simulink model "paper1_cs"  (R2021b)
settings: Solver=ode4  StartTime=0.0  StopTime=120  FixedStep=1/20  RelTol=1e-3
PreLoadFcn:
  | mbxruntime.callbacks.PreLoadFcn(bdroot);
PostLoadFcn:
  | mbxruntime.callbacks.PostLoadFcn(bdroot);
InitFcn:
  | mbxruntime.callbacks.InitFcn(bdroot);
StartFcn:
  | mbxruntime.callbacks.StartFcn(bdroot);
StopFcn:
  | mbxruntime.callbacks.StopFcn(bdroot);
model workspace (MAT data in the model file):
  mbox_table : object (value not decoded)
  model_closed = 0
  sim_status = 0
undefined symbols (not defined in the file): DiscIntNeverNeededParam
libraries: PreScanSimulinkLibrary x12, Solver_SF x6, simulink x1
(part 1 of 3)
CloseFcn:
  | mbxruntime.callbacks.CloseFcn(bdroot);
settings Model: Creator=PRESCAN  LastModifiedBy=Neutrin
settings SolverCC: AlgebraicLoopSolver=TrustRegion
settings DataIOCC: LimitDataPoints=on  SaveFormat=Array  SignalLoggingSaveFormat=ModelDataLogs  ReturnWorkspaceOutputs=off
settings OptimizationCC: ExpressionDepthLimit=2147483647  InitFltsAndDblsToZero=on  LifeSpan=inf
settings DebuggingCC: SaveWithParameterizedLinksMsg=none  UnderspecifiedInitializationDetection=Classic  MergeDetectMultiDrivingBlocksExec=none  SignalResolutionControl=TryResolveAllWithWarning  MultiTaskDSMMsg=warning  MultiTaskCondExecSysMsg=none  FcnCallInpInsideContextMsg=warning  StateNameClashWarn=warning  SFUnexpectedBacktrackingDiag=warning  SFNoUnconditionalDefaultTransitionDiag=warning  SFExecutionAtInitializationDiag=none  SFMachineParentedDataDiag=warning  ArithmeticOperatorsInVariantConditions=warning
settings HardwareCC: ProdBitPerPointer=32  ProdBitPerSizeT=32  ProdBitPerPtrDiffT=32  ProdLargestAtomicFloat=None  ProdIntDivRoundTo=Undefined  ProdEndianess=Unspecified  ProdWordSize=32  ProdHWDeviceType=32-bit Generic
settings ModelReferenceCC: UpdateModelReferenceTargets=IfOutOfDate  PropagateSignalLabelsOutOfModel=off
settings SFSimCC: SimUseLocalCustomCode=off  SimParseCustomCode=off  CustomCodeUndefinedFunction=UseInterfaceOnly
settings SFSimCC: SimCustomHeaderCode=|
  | #include "prescan.h"
  | #include "prescan_platform.h"
settings RTWCC: RTWUseLocalCustomCode=off
settings CodeAppCC: StateflowObjectComments=on
settings GRTTargetCC: TargetFcnLib=ansi_tfl_tmw.mat  TargetLangStandard=C89/C90 (ANSI)  CombineOutputUpdateFcns=off  GRTInterface=on
settings ConfigComp: CovMetricSettings=dw  CovSaveCumulativeToWorkspaceVar=on  CovSaveSingleToWorkspaceVar=on  CovExternalEMLEnable=off

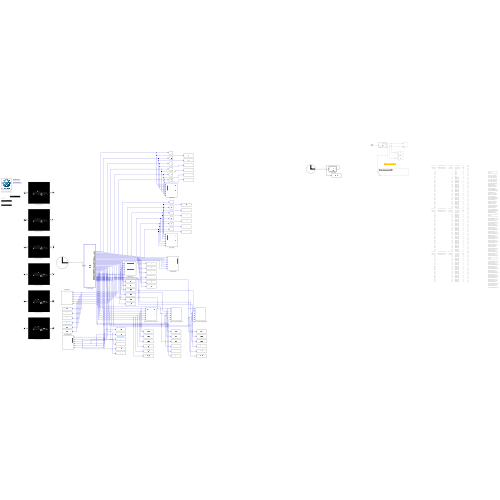
[thumbnail: Simulink's stored preview of the top-level diagram]
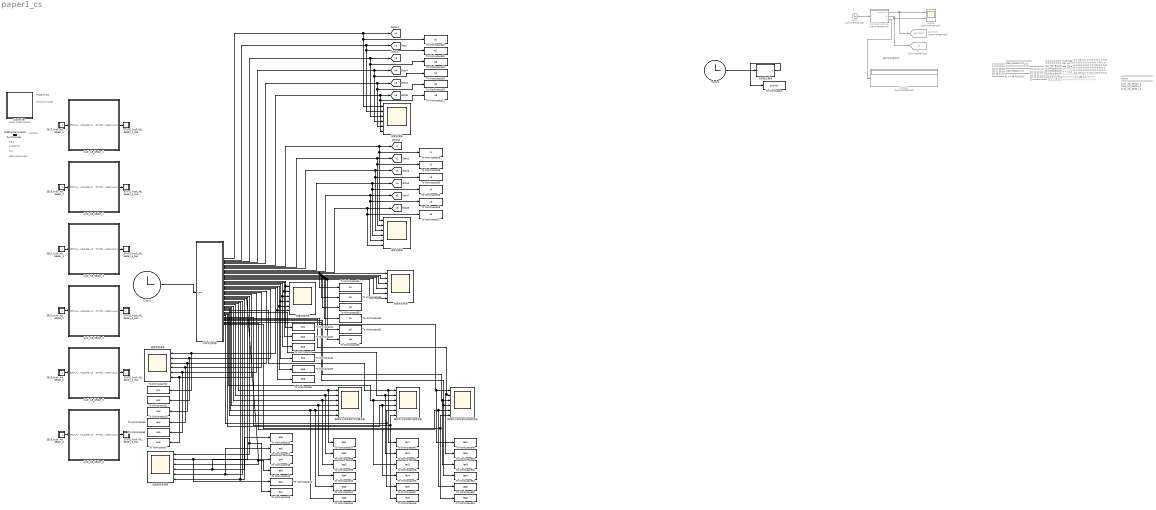
== system paper1_cs ==
  note: 虚拟领导者模块
  note: Regenerate
  note: Simulink Mode
  note: Open Useful Blocks
  note: 8.5.0
  note: Version:
  note: Author(s):
  note: N.A.
  note: Descriptive text:
  note: ======
      | Num ID
      | ======
      | 3
      | 11
      | 12
      | 13
      | 14
      | 15
      | 17
      | 19
      | 18
      | 25
      | 26
      | 27
      | 28
      | 29
      | 30
      | 32
      | 33
      | 34
      | 35
      | 36
      | 37
      | 38
      | 39
      | 40
      | 41
      | 42
      | 43
      | 44
      | 45
      | 46
      | ======
      | Num ID
      | ======
      | 31
      | 47
      | 48
      | 49
      | 50
      | 51
      | 52
      | 53
      | 54
      | 55
      | 56
      | 57
      | 58
      | 59
      | 60
      | 61
      | 62
      | 63
      | 64
      | 65
      | 66
      | 24
      | 67
      | 68
      | 20
      | 21
      | 22
      | 69
      | 70
      | 71
      | ======
      | Num ID
      | ======
      | 72
      | 73
      | 74
      | 75
      | 76
      | 77
      | 78
      | 79
      | 80
      | 81
      | 82
      | 83
      | 84
      | 85
      | 86
      | 87
      | 88
      | 89
      | 90
      | 91
      | 92
  note: =============
      | OBU-Beacon ID
      | =============
      |
      |
      |
      |
      |
      |
      |
      |
      |
      |
      |
      |
      |
      |
      |
      |
      |
      |
      |
      |
      |
      |
      |
      |
      |
      |
      |
      |
      |
      |
      | =============
      | OBU-Beacon ID
      | =============
      |
      |
      |
      |
      |
      |
      |
      |
      |
      |
      |
      |
      |
      |
      |
      |
      |
      |
      |
      |
      |
      |
      |
      |
      |
      |
      |
      |
      |
      |
      | =============
      | OBU-Beacon ID
      | =============
  note: =======
      | Type ID
      | =======
      | 1
      | 1
      | 1
      | 1
      | 1
      | 1
      | 12
      | 12
      | 12
      | 12
      | 12
      | 12
      | 12
      | 12
      | 12
      | 12
      | 12
      | 12
      | 12
      | 12
      | 12
      | 12
      | 12
      | 12
      | 12
      | 12
      | 12
      | 12
      | 12
      | 12
      | =======
      | Type ID
      | =======
      | 12
      | 12
      | 12
      | 12
      | 12
      | 12
      | 12
      | 12
      | 12
      | 12
      | 12
      | 12
      | 12
      | 12
      | 12
      | 12
      | 12
      | 12
      | 12
      | 12
      | 12
      | 12
      | 12
      | 12
      | 12
      | 12
      | 12
      | 12
      | 12
      | 12
      | =======
      | Type ID
      | =======
      | 12
      | 12
      | 12
      | 12
      | 12
      | 12
      | 12
      | 12
      | 12
      | 12
      | 12
      | 12
      | 12
      | 12
      | 12
      | 12
      | 12
      | 12
      | 12
      | 12
      | 12
  note: ========
      | Type Tag
      | ========
      | Car
      | Car
      | Car
      | Car
      | Car
      | Car
      | Building
      | Building
      | Building
      | Building
      | Building
      | Building
      | Building
      | Building
      | Building
      | Building
      | Building
      | Building
      | Building
      | Building
      | Building
      | Building
      | Building
      | Building
      | Building
      | Building
      | Building
      | Building
      | Building
      | Building
      | ========
      | Type Tag
      | ========
      | Building
      | Building
      | Building
      | Building
      | Building
      | Building
      | Building
      | Building
      | Building
      | Building
      | Building
      | Building
      | Building
      | Building
      | Building
      | Building
      | Building
      | Building
      | Building
      | Building
      | Building
      | Building
      | Building
      | Building
      | Building
      | Building
      | Building
      | Building
      | Building
      | Building
      | ========
      | Type Tag
      | ========
      | Building
      | Building
      | Building
      | Building
      | Building
      | Building
      | Building
      | Building
      | Building
      | Building
      | Building
      | Building
      | Building
      | Building
      | Building
      | Building
      | Building
      | Building
      | Building
      | Building
      | Building
  note: ==
      | SD
      | ==
      | Y
      | Y
      | Y
      | Y
      | Y
      | Y
      | Y
      | Y
      | Y
      | Y
      | Y
      | Y
      | Y
      | Y
      | Y
      | Y
      | Y
      | Y
      | Y
      | Y
      | Y
      | Y
      | Y
      | Y
      | Y
      | Y
      | Y
      | Y
      | Y
      | Y
      | ==
      | SD
      | ==
      | Y
      | Y
      | Y
      | Y
      | Y
      | Y
      | Y
      | Y
      | Y
      | Y
      | Y
      | Y
      | Y
      | Y
      | Y
      | Y
      | Y
      | Y
      | Y
      | Y
      | Y
      | Y
      | Y
      | Y
      | Y
      | Y
      | Y
      | Y
      | Y
      | Y
      | ==
      | SD
      | ==
      | Y
      | Y
      | Y
      | Y
      | Y
      | Y
      | Y
      | Y
      | Y
      | Y
      | Y
      | Y
      | Y
      | Y
      | Y
      | Y
      | Y
      | Y
      | Y
      | Y
      | Y
  note: ==
      | CD
      | ==
      | N
      | N
      | N
      | N
      | N
      | N
      | N
      | N
      | N
      | N
      | N
      | N
      | N
      | N
      | N
      | N
      | N
      | N
      | N
      | N
      | N
      | N
      | N
      | N
      | N
      | N
      | N
      | N
      | N
      | N
      | ==
      | CD
      | ==
      | N
      | N
      | N
      | N
      | N
      | N
      | N
      | N
      | N
      | N
      | N
      | N
      | N
      | N
      | N
      | N
      | N
      | N
      | N
      | N
      | N
      | N
      | N
      | N
      | N
      | N
      | N
      | N
      | N
      | N
      | ==
      | CD
      | ==
      | N
      | N
      | N
      | N
      | N
      | N
      | N
      | N
      | N
      | N
      | N
      | N
      | N
      | N
      | N
      | N
      | N
      | N
      | N
      | N
      | N
  note: ================
      | Name
      | ================
      | Audi_A8_Sedan_1
      | Audi_A8_Sedan_2
      | Audi_A8_Sedan_3
      | Audi_A8_Sedan_4
      | Audi_A8_Sedan_5
      | Audi_A8_Sedan_6
      | ApartmentBuilding_1
      | HouseModern_1
      | OfficeGreenTall_1
      | OfficeGreenTall_3
      | HouseModern_3
      | ApartmentBuilding_3
      | ApartmentBuilding_4
      | HouseModern_4
      | OfficeGreenTall_4
      | OfficeGreenTall_5
      | HouseModern_5
      | ApartmentBuilding_5
      | ApartmentBuilding_6
      | HouseModern_6
      | OfficeGreenTall_6
      | OfficeGreenTall_7
      | HouseModern_7
      | ApartmentBuilding_7
      | OfficeGreenTall_8
      | HouseModern_8
      | ApartmentBuilding_8
      | ApartmentBuilding_9
      | HouseModern_9
      | OfficeGreenTall_9
      | ================
      | Name
      | ================
      | ApartmentBuilding_10
      | HouseModern_10
      | OfficeGreenTall_10
      | ApartmentBuilding_11
      | HouseModern_11
      | OfficeGreenTall_11
      | ApartmentBuilding_12
      | HouseModern_12
      | OfficeGreenTall_12
      | ApartmentBuilding_13
      | HouseModern_13
      | OfficeGreenTall_13
      | ApartmentBuilding_14
      | HouseModern_14
      | OfficeGreenTall_14
      | ApartmentBuilding_15
      | HouseModern_15
      | OfficeGreenTall_15
      | ApartmentBuilding_16
      | HouseModern_16
      | OfficeGreenTall_16
      | OfficeGreenTall_2
      | HouseModern_2
      | ApartmentBuilding_2
      | OfficeGreenTall_17
      | HouseModern_17
      | ApartmentBuilding_17
      | OfficeGreenTall_18
      | HouseModern_18
      | ApartmentBuilding_18
      | ================
      | Name
      | ================
      | ApartmentBuilding_19
      | HouseModern_19
      | OfficeGreenTall_19
      | ApartmentBuilding_20
      | HouseModern_20
      | OfficeGreenTall_20
      | ApartmentBuilding_21
      | HouseModern_21
      | OfficeGreenTall_21
      | ApartmentBuilding_22
      | HouseModern_22
      | OfficeGreenTall_22
      | ApartmentBuilding_23
      | HouseModern_23
      | OfficeGreenTall_23
      | OfficeGreenTall_24
      | HouseModern_24
      | ApartmentBuilding_24
      | OfficeGreenTall_25
      | HouseModern_25
      | ApartmentBuilding_25
  Audi_A8_Sedan_1 : Subsystem  Tag=WorldObjectSubSystem  InitFcn=UniqueId = '64';
      mask init:
      | modelPath = GenericModelHelper.getGenericModelFilePath('ModelDepo','Vehicles\Audi_A8\Audi_A8.pgmb','d771622804618130053427da08a6d484');imagePath = GenericModelHelper.getCompilationPicture(modelPath, 'Audi_A8_HighPoly.png');
      mask Display: image(imread(imagePath));color('white');text(0, 0, ' ID=3\n')
  Audi_A8_Sedan_2 : Subsystem  Tag=WorldObjectSubSystem  InitFcn=UniqueId = '65';
      mask init: same as paper1_cs/Audi_A8_Sedan_1
      mask Display: image(imread(imagePath));color('white');text(0, 0, ' ID=11\n')
  Audi_A8_Sedan_3 : Subsystem  Tag=WorldObjectSubSystem  InitFcn=UniqueId = '66';
      mask init: same as paper1_cs/Audi_A8_Sedan_1
      mask Display: image(imread(imagePath));color('white');text(0, 0, ' ID=12\n')
  Audi_A8_Sedan_4 : Subsystem  Tag=WorldObjectSubSystem  InitFcn=UniqueId = '67';
      mask init: same as paper1_cs/Audi_A8_Sedan_1
      mask Display: image(imread(imagePath));color('white');text(0, 0, ' ID=13\n')
  Audi_A8_Sedan_5 : Subsystem  Tag=WorldObjectSubSystem  InitFcn=UniqueId = '68';
      mask init: same as paper1_cs/Audi_A8_Sedan_1
      mask Display: image(imread(imagePath));color('white');text(0, 0, ' ID=14\n')
  Audi_A8_Sedan_6 : Subsystem  Tag=WorldObjectSubSystem  InitFcn=UniqueId = '69';
      mask init: same as paper1_cs/Audi_A8_Sedan_1
      mask Display: image(imread(imagePath));color('white');text(0, 0, ' ID=15\n')
  Clock : Clock  Commented=on
  Clock1 : Clock
  Clock2 : Clock
  Controller : Subsystem  Description=FAA03037B41319C220BECF1B5D4CC9BCB680DCDF6B1D9774133C0D9A14409DD5  Priority=-1  LoadFcn=load PreScanControllerData  mask(PreScan Simulation Controller){prescanversion='8.5.0', ModelReferencing=off, TimeStep=1/20, ControlMode=0, PreScanExecutionMode=on, ControllerCount=0, ControllerIndex=0, ControllerOptions=''}
      mask prompts: prescanversion "PreScan Version"; ModelReferencing "Use Model Referencing"; TimeStep "Upload Period [s]"; ControlMode "Control Mode"; PreScanExecutionMode "Execution Mode"; ControllerCount "Controller Count"; ControllerIndex "Controller Index"; ControllerOptions "Controller Options"
      mask help:
      | Please do not remove this block from the compilation sheet,
      | as it connects the model to the PreScan environment.
      mask init:
      | model = bdroot(gcb);
      | ExperimentFile = mbxruntime.findExperimentFile(model,true); %relative path
      | 
      | [d1, d2, d3, prescandata] = prescan_Settings();
      | ModelDepo = fullfile(prescandata,'ModelDepo'); 
      | 
      | RTmode = mbxruntime.getRTMode(model);
      | 
      | SimulationMode = get_param(bdroot,'SimulationMode');
      | if strcmp(SimulationMode, 'rapid-accelerator')
      |     SimulationMode = 'external';
      | end
      | TargetName = get_param(bdroot,'SystemTargetFile');
      settings: ModelCloseFcn=assignin('base',['model_closed_' bdroot],true);
      mask Help: eval('openHelp(812)')
      mask Display: image(imread('prescanlogo.ico'))
  Display : Display  Commented=on
  MATLAB Function : MATLAB Function  Commented=on  TreatAsAtomicUnit=on
  PreScanTerminator : Subsystem  Tag=PreScanTerminator  Priority=999  LoadFcn=load PrescanTerminatorData  mask(PreScan Simulation Terminator){TimeStep=1/20}
      mask prompts: TimeStep "Upload Period [s]"
      mask help:
      | Please do not remove this block from the compilation sheet as it
      | connects the model to the PreScan environment.
      mask Help: eval('openHelp(812)')
      mask Display: image(imread('prescanlogo.ico'))
  SELF_Audi_A8_Sedan_1 : Subsystem  Tag=sensor/SelfPort  Priority=3  LoadFcn=load('PreScanSelfSensorData.mat')  mask(PreScan Source Block: SELF){}
      mask help:
      | The SELF port shows (state) information of the actor itself. The outputs are position in the experiment's axis system and the GPS coordinates, and the object's absolute velocity and compass heading.
      |
      | For more information, please click Help.
      settings: OpenFcn=open_system([gcb '/Sensor'],'mask')
      mask Help: eval('openHelp(462)')
      mask Display: image(imread('GPS.png'))
  SELF_Audi_A8_Sedan_2 : Subsystem  Tag=sensor/SelfPort  Priority=3  LoadFcn=load('PreScanSelfSensorData.mat')  mask(PreScan Source Block: SELF){}
      mask help:
      | The SELF port shows (state) information of the actor itself. The outputs are position in the experiment's axis system and the GPS coordinates, and the object's absolute velocity and compass heading.
      |
      | For more information, please click Help.
      settings: OpenFcn=open_system([gcb '/Sensor'],'mask')
      mask Help: eval('openHelp(462)')
      mask Display: image(imread('GPS.png'))
  SELF_Audi_A8_Sedan_3 : Subsystem  Tag=sensor/SelfPort  Priority=3  LoadFcn=load('PreScanSelfSensorData.mat')  mask(PreScan Source Block: SELF){}
      mask help:
      | The SELF port shows (state) information of the actor itself. The outputs are position in the experiment's axis system and the GPS coordinates, and the object's absolute velocity and compass heading.
      |
      | For more information, please click Help.
      settings: OpenFcn=open_system([gcb '/Sensor'],'mask')
      mask Help: eval('openHelp(462)')
      mask Display: image(imread('GPS.png'))
  SELF_Audi_A8_Sedan_4 : Subsystem  Tag=sensor/SelfPort  Priority=3  LoadFcn=load('PreScanSelfSensorData.mat')  mask(PreScan Source Block: SELF){}
      mask help:
      | The SELF port shows (state) information of the actor itself. The outputs are position in the experiment's axis system and the GPS coordinates, and the object's absolute velocity and compass heading.
      |
      | For more information, please click Help.
      settings: OpenFcn=open_system([gcb '/Sensor'],'mask')
      mask Help: eval('openHelp(462)')
      mask Display: image(imread('GPS.png'))
  SELF_Audi_A8_Sedan_5 : Subsystem  Tag=sensor/SelfPort  Priority=3  LoadFcn=load('PreScanSelfSensorData.mat')  mask(PreScan Source Block: SELF){}
      mask help:
      | The SELF port shows (state) information of the actor itself. The outputs are position in the experiment's axis system and the GPS coordinates, and the object's absolute velocity and compass heading.
      |
      | For more information, please click Help.
      settings: OpenFcn=open_system([gcb '/Sensor'],'mask')
      mask Help: eval('openHelp(462)')
      mask Display: image(imread('GPS.png'))
  SELF_Audi_A8_Sedan_6 : Subsystem  Tag=sensor/SelfPort  Priority=3  LoadFcn=load('PreScanSelfSensorData.mat')  mask(PreScan Source Block: SELF){}
      mask help:
      | The SELF port shows (state) information of the actor itself. The outputs are position in the experiment's axis system and the GPS coordinates, and the object's absolute velocity and compass heading.
      |
      | For more information, please click Help.
      settings: OpenFcn=open_system([gcb '/Sensor'],'mask')
      mask Help: eval('openHelp(462)')
      mask Display: image(imread('GPS.png'))
  STATE_Audi_A8_Sedan_1_bus : Subsystem  Tag=actuator/StatePort  Priority=0  LoadFcn=load('PreScanStateActuatorData.mat')  mask(PreScan Sink Block: State){}
      mask help:
      | The Actor State contains a vector signal of size (9x1), containing the following signals:
      |
      | -  Position    	(x,y,z)             	[m]
      | -  Velocity    	(vx,vy,vz)         	[m/s]
      | -  Angles       	(Roll, Pitch, Yaw)	[rad]
      |
      | The Actor state is defined in the global axis system.
      | The state is superponed on the Initial position defined in the GUI.
      |
      | For more information, please click Help.
      settings: OpenFcn=open_system([gcb '/Actuator'],'mask')
      mask Help: eval('openHelp(222)')
      mask Display: image(imread('State.png'))
  STATE_Audi_A8_Sedan_2_bus : Subsystem  Tag=actuator/StatePort  Priority=0  LoadFcn=load('PreScanStateActuatorData.mat')  mask(PreScan Sink Block: State){}
      mask help:
      | The Actor State contains a vector signal of size (9x1), containing the following signals:
      |
      | -  Position    	(x,y,z)             	[m]
      | -  Velocity    	(vx,vy,vz)         	[m/s]
      | -  Angles       	(Roll, Pitch, Yaw)	[rad]
      |
      | The Actor state is defined in the global axis system.
      | The state is superponed on the Initial position defined in the GUI.
      |
      | For more information, please click Help.
      settings: OpenFcn=open_system([gcb '/Actuator'],'mask')
      mask Help: eval('openHelp(222)')
      mask Display: image(imread('State.png'))
  STATE_Audi_A8_Sedan_3_bus : Subsystem  Tag=actuator/StatePort  Priority=0  LoadFcn=load('PreScanStateActuatorData.mat')  mask(PreScan Sink Block: State){}
      mask help:
      | The Actor State contains a vector signal of size (9x1), containing the following signals:
      |
      | -  Position    	(x,y,z)             	[m]
      | -  Velocity    	(vx,vy,vz)         	[m/s]
      | -  Angles       	(Roll, Pitch, Yaw)	[rad]
      |
      | The Actor state is defined in the global axis system.
      | The state is superponed on the Initial position defined in the GUI.
      |
      | For more information, please click Help.
      settings: OpenFcn=open_system([gcb '/Actuator'],'mask')
      mask Help: eval('openHelp(222)')
      mask Display: image(imread('State.png'))
  STATE_Audi_A8_Sedan_4_bus : Subsystem  Tag=actuator/StatePort  Priority=0  LoadFcn=load('PreScanStateActuatorData.mat')  mask(PreScan Sink Block: State){}
      mask help:
      | The Actor State contains a vector signal of size (9x1), containing the following signals:
      |
      | -  Position    	(x,y,z)             	[m]
      | -  Velocity    	(vx,vy,vz)         	[m/s]
      | -  Angles       	(Roll, Pitch, Yaw)	[rad]
      |
      | The Actor state is defined in the global axis system.
      | The state is superponed on the Initial position defined in the GUI.
      |
      | For more information, please click Help.
      settings: OpenFcn=open_system([gcb '/Actuator'],'mask')
      mask Help: eval('openHelp(222)')
      mask Display: image(imread('State.png'))
  STATE_Audi_A8_Sedan_5_bus : Subsystem  Tag=actuator/StatePort  Priority=0  LoadFcn=load('PreScanStateActuatorData.mat')  mask(PreScan Sink Block: State){}
      mask help:
      | The Actor State contains a vector signal of size (9x1), containing the following signals:
      |
      | -  Position    	(x,y,z)             	[m]
      | -  Velocity    	(vx,vy,vz)         	[m/s]
      | -  Angles       	(Roll, Pitch, Yaw)	[rad]
      |
      | The Actor state is defined in the global axis system.
      | The state is superponed on the Initial position defined in the GUI.
      |
      | For more information, please click Help.
      settings: OpenFcn=open_system([gcb '/Actuator'],'mask')
      mask Help: eval('openHelp(222)')
      mask Display: image(imread('State.png'))
  STATE_Audi_A8_Sedan_6_bus : Subsystem  Tag=actuator/StatePort  Priority=0  LoadFcn=load('PreScanStateActuatorData.mat')  mask(PreScan Sink Block: State){}
      mask help:
      | The Actor State contains a vector signal of size (9x1), containing the following signals:
      |
      | -  Position    	(x,y,z)             	[m]
      | -  Velocity    	(vx,vy,vz)         	[m/s]
      | -  Angles       	(Roll, Pitch, Yaw)	[rad]
      |
      | The Actor state is defined in the global axis system.
      | The state is superponed on the Initial position defined in the GUI.
      |
      | For more information, please click Help.
      settings: OpenFcn=open_system([gcb '/Actuator'],'mask')
      mask Help: eval('openHelp(222)')
      mask Display: image(imread('State.png'))
  Scope : Scope  Commented=on  NumInputPorts=2
  Synchronizer : Subsystem  Tag=PreScanSynchronizer  Priority=1  LoadFcn=load PrescanSynchronizeData  mask(PreScan Simulation Core Block){TimeStep=1/20}
      mask prompts: TimeStep "Timestep [s]"
      mask help:
      | Please do not remove this block from the PreScan compilation sheet,
      | as it contains essential configuration parameters for a PreScan simulation.
      settings: DeleteFcn=PreScanBlockDeleteFcn;
      mask Display: image(imread('prescanlogo.ico'))
  To Workspace : ToWorkspace  VariableName=simout  SaveFormat=Timeseries  SampleTime=-1
  To Workspace1 : ToWorkspace  VariableName=ep1  SaveFormat=Timeseries  SampleTime=-1
  To Workspace10 : ToWorkspace  VariableName=ev3  SaveFormat=Timeseries  SampleTime=-1
  To Workspace11 : ToWorkspace  VariableName=ev2  SaveFormat=Timeseries  SampleTime=-1
  To Workspace12 : ToWorkspace  VariableName=ev1  SaveFormat=Timeseries  SampleTime=-1
  To Workspace13 : ToWorkspace  VariableName=ea3  SaveFormat=Timeseries  SampleTime=-1
  To Workspace14 : ToWorkspace  VariableName=ea2  SaveFormat=Timeseries  SampleTime=-1
  To Workspace15 : ToWorkspace  VariableName=ea1  SaveFormat=Timeseries  SampleTime=-1
  To Workspace16 : ToWorkspace  VariableName=ea6  SaveFormat=Timeseries  SampleTime=-1
  To Workspace17 : ToWorkspace  VariableName=ea5  SaveFormat=Timeseries  SampleTime=-1
  To Workspace18 : ToWorkspace  VariableName=ea4  SaveFormat=Timeseries  SampleTime=-1
  To Workspace19 : ToWorkspace  VariableName=p4  SaveFormat=Timeseries  SampleTime=-1
  To Workspace2 : ToWorkspace  VariableName=ep2  SaveFormat=Timeseries  SampleTime=-1
  To Workspace20 : ToWorkspace  VariableName=p5  SaveFormat=Timeseries  SampleTime=-1
  To Workspace21 : ToWorkspace  VariableName=p6  SaveFormat=Timeseries  SampleTime=-1
  To Workspace22 : ToWorkspace  VariableName=p1  SaveFormat=Timeseries  SampleTime=-1
  To Workspace23 : ToWorkspace  VariableName=p2  SaveFormat=Timeseries  SampleTime=-1
  To Workspace24 : ToWorkspace  VariableName=p3  SaveFormat=Timeseries  SampleTime=-1
  To Workspace25 : ToWorkspace  VariableName=v4  SaveFormat=Timeseries  SampleTime=-1
  To Workspace26 : ToWorkspace  VariableName=v5  SaveFormat=Timeseries  SampleTime=-1
  To Workspace27 : ToWorkspace  VariableName=v6  SaveFormat=Timeseries  SampleTime=-1
  To Workspace28 : ToWorkspace  VariableName=v1  SaveFormat=Timeseries  SampleTime=-1
  To Workspace29 : ToWorkspace  VariableName=v2  SaveFormat=Timeseries  SampleTime=-1
  To Workspace3 : ToWorkspace  VariableName=ep3  SaveFormat=Timeseries  SampleTime=-1
  To Workspace30 : ToWorkspace  VariableName=v3  SaveFormat=Timeseries  SampleTime=-1
  To Workspace31 : ToWorkspace  VariableName=a4  SaveFormat=Timeseries  SampleTime=-1
  To Workspace32 : ToWorkspace  VariableName=a5  SaveFormat=Timeseries  SampleTime=-1
  To Workspace33 : ToWorkspace  VariableName=a6  SaveFormat=Timeseries  SampleTime=-1
  To Workspace34 : ToWorkspace  VariableName=a1  SaveFormat=Timeseries  SampleTime=-1
  To Workspace35 : ToWorkspace  VariableName=a2  SaveFormat=Timeseries  SampleTime=-1
  To Workspace36 : ToWorkspace  VariableName=a3  SaveFormat=Timeseries  SampleTime=-1
  To Workspace37 : ToWorkspace  VariableName=lep1  SaveFormat=Timeseries  SampleTime=-1
  To Workspace38 : ToWorkspace  VariableName=lep2  SaveFormat=Timeseries  SampleTime=-1
  To Workspace39 : ToWorkspace  VariableName=lep3  SaveFormat=Timeseries  SampleTime=-1
  To Workspace4 : ToWorkspace  VariableName=ep4  SaveFormat=Timeseries  SampleTime=-1
  To Workspace40 : ToWorkspace  VariableName=lep4  SaveFormat=Timeseries  SampleTime=-1
  To Workspace41 : ToWorkspace  VariableName=lep5  SaveFormat=Timeseries  SampleTime=-1
  To Workspace42 : ToWorkspace  VariableName=lep6  SaveFormat=Timeseries  SampleTime=-1
  To Workspace43 : ToWorkspace  VariableName=lev1  SaveFormat=Timeseries  SampleTime=-1
  To Workspace44 : ToWorkspace  VariableName=lev2  SaveFormat=Timeseries  SampleTime=-1
  To Workspace45 : ToWorkspace  VariableName=lev3  SaveFormat=Timeseries  SampleTime=-1
  To Workspace46 : ToWorkspace  VariableName=lev4  SaveFormat=Timeseries  SampleTime=-1
  To Workspace47 : ToWorkspace  VariableName=lev5  SaveFormat=Timeseries  SampleTime=-1
  To Workspace48 : ToWorkspace  VariableName=lev6  SaveFormat=Timeseries  SampleTime=-1
  To Workspace49 : ToWorkspace  VariableName=lea1  SaveFormat=Timeseries  SampleTime=-1
  To Workspace5 : ToWorkspace  VariableName=ep5  SaveFormat=Timeseries  SampleTime=-1
  To Workspace50 : ToWorkspace  VariableName=lea2  SaveFormat=Timeseries  SampleTime=-1
  To Workspace51 : ToWorkspace  VariableName=lea3  SaveFormat=Timeseries  SampleTime=-1
  To Workspace52 : ToWorkspace  VariableName=lea4  SaveFormat=Timeseries  SampleTime=-1
  To Workspace53 : ToWorkspace  VariableName=lea5  SaveFormat=Timeseries  SampleTime=-1
  To Workspace54 : ToWorkspace  VariableName=lea6  SaveFormat=Timeseries  SampleTime=-1
  To Workspace6 : ToWorkspace  VariableName=ep6  SaveFormat=Timeseries  SampleTime=-1
  To Workspace7 : ToWorkspace  VariableName=ev6  SaveFormat=Timeseries  SampleTime=-1
  To Workspace8 : ToWorkspace  VariableName=ev5  SaveFormat=Timeseries  SampleTime=-1
  To Workspace9 : ToWorkspace  VariableName=ev4  SaveFormat=Timeseries  SampleTime=-1
  position0 : Goto  Commented=on  GotoTag=position0  TagVisibility=global
  v0 : Goto  Commented=on  GotoTag=v0  TagVisibility=global
  位置监视器 : Scope  NumInputPorts=6
  位置观测误差 : Scope  NumInputPorts=6
  分布式控制器 : MATLAB Function  TreatAsAtomicUnit=on
  加速度监视器 : Scope  NumInputPorts=6
  加速度观测误差 : Scope  NumInputPorts=6
  时序验证模块 : MATLAB Function  TreatAsAtomicUnit=on
  跟随车与领导者的加速度误差 : Scope  NumInputPorts=6
  跟随车与领导者的状位置误差 : Scope  NumInputPorts=6
  跟随车与领导者的速度误差 : Scope  NumInputPorts=6
  速度监视器 : Scope  NumInputPorts=6
  速度观测误差 : Scope  NumInputPorts=6
  tag scope: v1=global, v2=global, v3=global, v4=global, v5=global, v6=global, x1=global, x2=global, x3=global, x4=global, x5=global, x6=global
  wires:
  Clock/1 -> MATLAB Function/1("t ")
  MATLAB Function/2(v0) -> v0/1, Scope/2
  MATLAB Function/1(position0) -> position0/1, Scope/1
  MATLAB Function/3(t) -> Display/1
  Clock1/1 -> 分布式控制器/1(time)
  时序验证模块/1(y) -> To Workspace/1
  Clock2/1 -> 时序验证模块/1(t)
  Audi_A8_Sedan_1/1(STATE_Audi_A8_Sedan_1_bus) -> STATE_Audi_A8_Sedan_1_bus/1(STATE_Audi_A8_Sedan_1_bus)
  SELF_Audi_A8_Sedan_1/1(SELF_Audi_A8_Sedan_1) -> Audi_A8_Sedan_1/1(SELF_Audi_A8_Sedan_1)
  Audi_A8_Sedan_2/1(STATE_Audi_A8_Sedan_2_bus) -> STATE_Audi_A8_Sedan_2_bus/1(STATE_Audi_A8_Sedan_2_bus)
  SELF_Audi_A8_Sedan_2/1(SELF_Audi_A8_Sedan_2) -> Audi_A8_Sedan_2/1(SELF_Audi_A8_Sedan_2)
  Audi_A8_Sedan_3/1(STATE_Audi_A8_Sedan_3_bus) -> STATE_Audi_A8_Sedan_3_bus/1(STATE_Audi_A8_Sedan_3_bus)
  SELF_Audi_A8_Sedan_3/1(SELF_Audi_A8_Sedan_3) -> Audi_A8_Sedan_3/1(SELF_Audi_A8_Sedan_3)
  Audi_A8_Sedan_4/1(STATE_Audi_A8_Sedan_4_bus) -> STATE_Audi_A8_Sedan_4_bus/1(STATE_Audi_A8_Sedan_4_bus)
  SELF_Audi_A8_Sedan_4/1(SELF_Audi_A8_Sedan_4) -> Audi_A8_Sedan_4/1(SELF_Audi_A8_Sedan_4)
  Audi_A8_Sedan_5/1(STATE_Audi_A8_Sedan_5_bus) -> STATE_Audi_A8_Sedan_5_bus/1(STATE_Audi_A8_Sedan_5_bus)
  SELF_Audi_A8_Sedan_5/1(SELF_Audi_A8_Sedan_5) -> Audi_A8_Sedan_5/1(SELF_Audi_A8_Sedan_5)
  Audi_A8_Sedan_6/1(STATE_Audi_A8_Sedan_6_bus) -> STATE_Audi_A8_Sedan_6_bus/1(STATE_Audi_A8_Sedan_6_bus)
  SELF_Audi_A8_Sedan_6/1(SELF_Audi_A8_Sedan_6) -> Audi_A8_Sedan_6/1(SELF_Audi_A8_Sedan_6)
  分布式控制器/1(p1) -> To Workspace22/1, 位置监视器/1, [x1]
  分布式控制器/2(p2) -> To Workspace23/1, 位置监视器/2, [x2]
  分布式控制器/3(p3) -> To Workspace24/1, 位置监视器/3, [x3]
  分布式控制器/4(p4) -> To Workspace19/1, 位置监视器/4, [x4]
  分布式控制器/5(p5) -> To Workspace20/1, 位置监视器/5, [x5]
  分布式控制器/6(p6) -> To Workspace21/1, 位置监视器/6, [x6]
  分布式控制器/7(v1) -> To Workspace28/1, 速度监视器/1, [v1]
  分布式控制器/8(v2) -> To Workspace29/1, 速度监视器/2, [v2]
  分布式控制器/9(v3) -> 速度监视器/3, To Workspace30/1, [v3]
  分布式控制器/10(v4) -> To Workspace25/1, 速度监视器/4, [v4]
  分布式控制器/11(v5) -> [v5], To Workspace26/1, 速度监视器/5
  分布式控制器/12(v6) -> To Workspace27/1, 速度监视器/6, [v6]
  分布式控制器/13(as1) -> 加速度监视器/1, To Workspace34/1
  分布式控制器/14(as2) -> To Workspace35/1, 加速度监视器/2
  分布式控制器/15(as3) -> To Workspace36/1, 加速度监视器/3
  分布式控制器/16(as4) -> To Workspace31/1, 加速度监视器/4
  分布式控制器/17(as5) -> To Workspace32/1, 加速度监视器/5
  分布式控制器/18(as6) -> To Workspace33/1, 加速度监视器/6
  分布式控制器/19(ep1) -> To Workspace1/1, 位置观测误差/1
  分布式控制器/20(ep2) -> To Workspace2/1, 位置观测误差/2
  分布式控制器/21(ep3) -> To Workspace3/1, 位置观测误差/3
  分布式控制器/22(ep4) -> To Workspace4/1, 位置观测误差/4
  分布式控制器/23(ep5) -> To Workspace5/1, 位置观测误差/5
  分布式控制器/24(ep6) -> To Workspace6/1, 位置观测误差/6
  分布式控制器/25(ev1) -> To Workspace12/1, 速度观测误差/1
  分布式控制器/26(ev2) -> To Workspace11/1, 速度观测误差/2
  分布式控制器/27(ev3) -> To Workspace10/1, 速度观测误差/3
  分布式控制器/28(ev4) -> To Workspace9/1, 速度观测误差/4
  分布式控制器/29(ev5) -> To Workspace8/1, 速度观测误差/5
  分布式控制器/30(ev6) -> To Workspace7/1, 速度观测误差/6
  分布式控制器/31(ea1) -> 加速度观测误差/1, To Workspace15/1
  分布式控制器/32(ea2) -> 加速度观测误差/2, To Workspace14/1
  分布式控制器/33(ea3) -> 加速度观测误差/3, To Workspace13/1
  分布式控制器/34(ea4) -> 加速度观测误差/4, To Workspace18/1
  分布式控制器/35(ea5) -> 加速度观测误差/5, To Workspace17/1
  分布式控制器/36(ea6) -> 加速度观测误差/6, To Workspace16/1
  分布式控制器/37(lep1) -> To Workspace37/1, 跟随车与领导者的状位置误差/1
  分布式控制器/38(lep2) -> To Workspace38/1, 跟随车与领导者的状位置误差/2
  分布式控制器/39(lep3) -> To Workspace39/1, 跟随车与领导者的状位置误差/3
  分布式控制器/40(lep4) -> To Workspace40/1, 跟随车与领导者的状位置误差/4
  分布式控制器/41(lep5) -> To Workspace42/1, To Workspace41/1, 跟随车与领导者的状位置误差/5
  分布式控制器/42(lep6) -> 跟随车与领导者的状位置误差/6
  分布式控制器/43(lev1) -> To Workspace43/1, 跟随车与领导者的速度误差/1
  分布式控制器/44(lev2) -> To Workspace44/1, 跟随车与领导者的速度误差/2
  分布式控制器/45(lev3) -> To Workspace45/1, 跟随车与领导者的速度误差/3
  分布式控制器/46(lev4) -> To Workspace46/1, 跟随车与领导者的速度误差/4
  分布式控制器/47(lev5) -> 跟随车与领导者的速度误差/5, To Workspace47/1
  分布式控制器/48(lev6) -> 跟随车与领导者的速度误差/6, To Workspace48/1
  分布式控制器/49(lea1) -> To Workspace49/1, 跟随车与领导者的加速度误差/1
  分布式控制器/50(lea2) -> To Workspace50/1, 跟随车与领导者的加速度误差/2
  分布式控制器/51(lea3) -> To Workspace51/1, 跟随车与领导者的加速度误差/3
  分布式控制器/52(lea4) -> To Workspace52/1, 跟随车与领导者的加速度误差/4
  分布式控制器/53(lea5) -> 跟随车与领导者的加速度误差/5, To Workspace53/1
  分布式控制器/54(lea6) -> To Workspace54/1, 跟随车与领导者的加速度误差/6

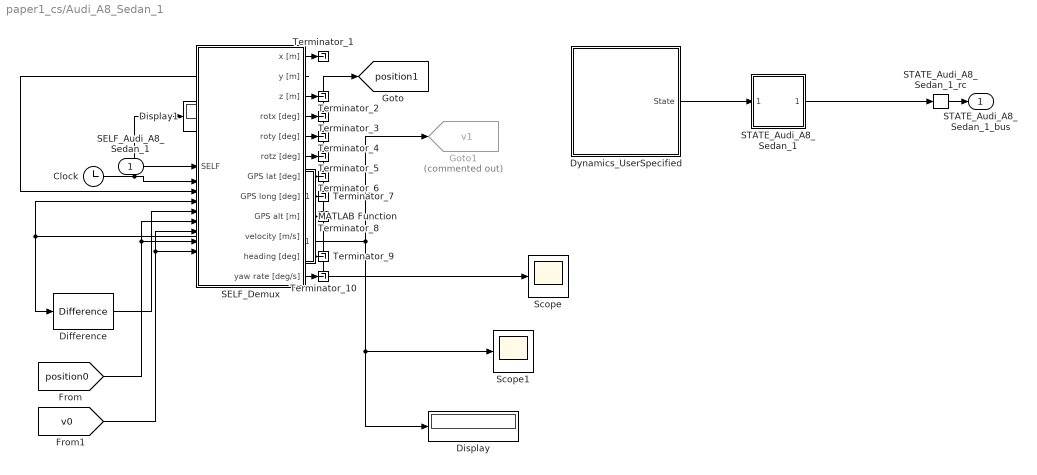
== system paper1_cs/Audi_A8_Sedan_1 ==
  SELF_Audi_A8_Sedan_1 : Inport  Tag=inport/SelfPort  OutDataTypeStr=Bus: PRESCAN_SELFSENSORDATA  PortDimensions=1  SampleTime=1/20  BusOutputAsStruct=on
  Clock : Clock
  Difference : simulink/Discrete/Difference  ICPrevInput=0.0  OutMin=[]  OutMax=[]  OutDataType=fixdt(1, 16)  OutScaling=2^-10  DoSatur=off
  Display : Display
  Display1 : Display
  Dynamics_UserSpecified : Subsystem  Tag=UserSpecified_Subsys  Description=..\..\..\DynamicMode\Extensions\Simulink\CarSim_VehicleDynamics.mdl  mask(User specified subsystem){update=off, sourcefilename=..\..\..\DynamicMode\Extensions\Simulink\CarSim_VehicleDynamics.mdl}
      mask prompts: update "Update (default: not checked)"; sourcefilename "Source file name"
      mask help:
      | A User-specified model may be selected as Controller or Dynamics of the vehicle. PreScan will copy the contents of the User-specified model into the user-specified model block.
      |
      | If update checkbox is checked the current user-specified model block will be deleted and will be REPLACED by (new) user specified model blocks. So, the current user specified model elements will be lost.
      |
      | Warning: If a new user-specified model is selected in the GUI, the user-specified model will be replaced.
      settings: DeleteFcn=PreScanBlockDeleteFcn;
      mask Help: eval('openHelp(227)')
      mask Display: userSpecifiedDynamics_mask_display();
  Goto1 : Goto  Commented=on  GotoTag=v1  TagVisibility=global
  MATLAB Function : MATLAB Function  TreatAsAtomicUnit=on
  SELF_Demux : Subsystem  Tag=demux/SelfPort  mask(PreScan Demux Block:){}
      mask help:
      | The SELF port shows (state) information of the actor itself. The outputs are position in the experiment's axis system and the GPS coordinates, and the object's absolute velocity and compass heading.
      |
      | For more information, please click Help.
      settings: DeleteFcn=PreScanBlockDeleteFcn;
      mask Help: eval('openHelp(462)')
      mask Display:
      | port_label('output',1,'x [m]')
      | port_label('output',2,'y [m]')
      | port_label('output',3,'z [m]','texmode','on')
      | port_label('output',4,'Rotx [deg]','texmode','on')
      | port_label('output',5,'Roty [deg]','texmode','on')
      | port_label('output',6,'Rotz [deg]','texmode','on')
      | port_label('output',7,'GPS lat [deg]','texmode','on')
      | port_label('output',8,'GPS long [deg]','texmode','on')
      | port_label('output',9,'GPS alt [m]','texmode','on')
      | port_label('output',10,'Velocity [m/s]')
      | port_label('output',11,'Heading [deg]')
      | port_label('output',12,'Yaw rate [deg/s]')
  STATE_Audi_A8_Sedan_1 : Subsystem  Tag=mux/StatePort  Priority=0  LoadFcn=load PrescanStateActuatorData  mask(PreScan Sink Block: State){x0=120, y0=85, z0=0.55, Roll0=0, Pitch0=0, Yaw0=0, TimeStep=1/20}
      mask prompts: x0 "Ini x-position VEHICLE wrt GLOBAL axis system [m]"; y0 "Ini y-position VEHICLE wrt GLOBAL axis system [m]"; z0 "Ini z-position VEHICLE wrt GLOBAL axis system [m]"; Roll0 "Ini roll-angle BODY wrt VEHICLE axis system [deg]"; Pitch0 "Ini pitch-angle BODY wrt VEHICLE axis system [deg]"; Yaw0 "Ini yaw-angle VEHICLE wrt GLOBAL axis system [deg]"; TimeStep "Auto-Assigned: Upload Period [s]"
      mask help:
      | The Actor State contains a vector signal of size (9x1), containing the following signals:
      |
      | -  Position                  (x,y,z)                                     [m]
      | -  Velocity                  (vx,vy,vz)                               [m/s]
      | -  Angles                    (Roll, Pitch, Yaw)                   [rad]
      |
      | The Actor state is defined in the global axis system.
      | The state is superponed on the Initial position defined in the GUI.
      |
      | For more information, please click Help.
      settings: DeleteFcn=PreScanBlockDeleteFcn;
      mask Help: eval('openHelp(222)')
      mask Display: image(imread('State.png'))
  STATE_Audi_A8_Sedan_1_rc : RateTransition  Tag=mux_rc/StatePort  OutPortSampleTimeOpt=Inherit
  Scope : Scope
  Scope1 : Scope
  Terminator_{1..10} (10 alike) : Terminator
  STATE_Audi_A8_Sedan_1_bus : Outport  Tag=outport/StatePort  OutDataTypeStr=Bus: PRESCAN_STATEACTUATORDATA  PortDimensions=1  SampleTime=1/20
  tag scope: position1=global
  wires:
  SELF_Demux/2(y [m]) -> MATLAB Function/2(p)
  SELF_Demux/10(velocity [m/s]) -> MATLAB Function/3(v), Difference/1
  MATLAB Function/1(position1) -> Scope/1, [position1]
  MATLAB Function/2(v1) -> Goto1/1, Scope1/1, Display/1
  Clock/1 -> Display1/1, MATLAB Function/1(t)
  Difference/1 -> MATLAB Function/4(a)
  [position0] -> MATLAB Function/7(position2), MATLAB Function/5(position0)
  [v0] -> MATLAB Function/8(v2), MATLAB Function/6(v0)
  STATE_Audi_A8_Sedan_1_rc/1 -> STATE_Audi_A8_Sedan_1_bus/1
  STATE_Audi_A8_Sedan_1/1(StateBus) -> STATE_Audi_A8_Sedan_1_rc/1
  SELF_Audi_A8_Sedan_1/1 -> SELF_Demux/1(SELF)
  Dynamics_UserSpecified/1(State) -> STATE_Audi_A8_Sedan_1/1(State)
  SELF_Demux/1(x [m]) -> Terminator_1/1
  SELF_Demux/3(z [m]) -> Terminator_2/1
  SELF_Demux/4(rotx [deg]) -> Terminator_3/1
  SELF_Demux/5(roty [deg]) -> Terminator_4/1
  SELF_Demux/6(rotz [deg]) -> Terminator_5/1
  SELF_Demux/7(GPS lat [deg]) -> Terminator_6/1
  SELF_Demux/8(GPS long [deg]) -> Terminator_7/1
  SELF_Demux/9(GPS alt [m]) -> Terminator_8/1
  SELF_Demux/11(heading [deg]) -> Terminator_9/1
  SELF_Demux/12(yaw rate [deg/s]) -> Terminator_10/1

== system paper1_cs/Audi_A8_Sedan_2 ==
  SELF_Audi_A8_Sedan_2 : Inport  Tag=inport/SelfPort  OutDataTypeStr=Bus: PRESCAN_SELFSENSORDATA  PortDimensions=1  SampleTime=1/20  BusOutputAsStruct=on
  Dynamics_UserSpecified : Subsystem  Tag=UserSpecified_Subsys  Description=..\..\..\DynamicMode\Extensions\Simulink\CarSim_VehicleDynamics.mdl  mask(User specified subsystem){update=off, sourcefilename=..\..\..\DynamicMode\Extensions\Simulink\CarSim_VehicleDynamics.mdl}
      mask prompts: update "Update (default: not checked)"; sourcefilename "Source file name"
      mask help:
      | A User-specified model may be selected as Controller or Dynamics of the vehicle. PreScan will copy the contents of the User-specified model into the user-specified model block.
      |
      | If update checkbox is checked the current user-specified model block will be deleted and will be REPLACED by (new) user specified model blocks. So, the current user specified model elements will be lost.
      |
      | Warning: If a new user-specified model is selected in the GUI, the user-specified model will be replaced.
      settings: DeleteFcn=PreScanBlockDeleteFcn;
      mask Help: eval('openHelp(227)')
      mask Display: userSpecifiedDynamics_mask_display();
  SELF_Demux : Subsystem  Tag=demux/SelfPort  mask(PreScan Demux Block:){}
      mask help:
      | The SELF port shows (state) information of the actor itself. The outputs are position in the experiment's axis system and the GPS coordinates, and the object's absolute velocity and compass heading.
      |
      | For more information, please click Help.
      settings: DeleteFcn=PreScanBlockDeleteFcn;
      mask Help: eval('openHelp(462)')
      mask Display:
      | port_label('output',1,'x [m]')
      | port_label('output',2,'y [m]')
      | port_label('output',3,'z [m]','texmode','on')
      | port_label('output',4,'Rotx [deg]','texmode','on')
      | port_label('output',5,'Roty [deg]','texmode','on')
      | port_label('output',6,'Rotz [deg]','texmode','on')
      | port_label('output',7,'GPS lat [deg]','texmode','on')
      | port_label('output',8,'GPS long [deg]','texmode','on')
      | port_label('output',9,'GPS alt [m]','texmode','on')
      | port_label('output',10,'Velocity [m/s]')
      | port_label('output',11,'Heading [deg]')
      | port_label('output',12,'Yaw rate [deg/s]')
  STATE_Audi_A8_Sedan_2 : Subsystem  Tag=mux/StatePort  Priority=0  LoadFcn=load PrescanStateActuatorData  mask(PreScan Sink Block: State){x0=100, y0=85, z0=0.55, Roll0=0, Pitch0=0, Yaw0=0, TimeStep=1/20}
      mask prompts: x0 "Ini x-position VEHICLE wrt GLOBAL axis system [m]"; y0 "Ini y-position VEHICLE wrt GLOBAL axis system [m]"; z0 "Ini z-position VEHICLE wrt GLOBAL axis system [m]"; Roll0 "Ini roll-angle BODY wrt VEHICLE axis system [deg]"; Pitch0 "Ini pitch-angle BODY wrt VEHICLE axis system [deg]"; Yaw0 "Ini yaw-angle VEHICLE wrt GLOBAL axis system [deg]"; TimeStep "Auto-Assigned: Upload Period [s]"
      mask help:
      | The Actor State contains a vector signal of size (9x1), containing the following signals:
      |
      | -  Position                  (x,y,z)                                     [m]
      | -  Velocity                  (vx,vy,vz)                               [m/s]
      | -  Angles                    (Roll, Pitch, Yaw)                   [rad]
      |
      | The Actor state is defined in the global axis system.
      | The state is superponed on the Initial position defined in the GUI.
      |
      | For more information, please click Help.
      settings: DeleteFcn=PreScanBlockDeleteFcn;
      mask Help: eval('openHelp(222)')
      mask Display: image(imread('State.png'))
  STATE_Audi_A8_Sedan_2_rc : RateTransition  Tag=mux_rc/StatePort  OutPortSampleTimeOpt=Inherit
  Terminator_{1..12} (12 alike) : Terminator
  STATE_Audi_A8_Sedan_2_bus : Outport  Tag=outport/StatePort  OutDataTypeStr=Bus: PRESCAN_STATEACTUATORDATA  PortDimensions=1  SampleTime=1/20
  wires:
  STATE_Audi_A8_Sedan_2_rc/1 -> STATE_Audi_A8_Sedan_2_bus/1
  STATE_Audi_A8_Sedan_2/1(StateBus) -> STATE_Audi_A8_Sedan_2_rc/1
  SELF_Audi_A8_Sedan_2/1 -> SELF_Demux/1(SELF)
  Dynamics_UserSpecified/1(State) -> STATE_Audi_A8_Sedan_2/1(State)
  SELF_Demux/1(x [m]) -> Terminator_1/1
  SELF_Demux/2(y [m]) -> Terminator_2/1
  SELF_Demux/3(z [m]) -> Terminator_3/1
  SELF_Demux/4(rotx [deg]) -> Terminator_4/1
  SELF_Demux/5(roty [deg]) -> Terminator_5/1
  SELF_Demux/6(rotz [deg]) -> Terminator_6/1
  SELF_Demux/7(GPS lat [deg]) -> Terminator_7/1
  SELF_Demux/8(GPS long [deg]) -> Terminator_8/1
  SELF_Demux/9(GPS alt [m]) -> Terminator_9/1
  SELF_Demux/10(velocity [m/s]) -> Terminator_10/1
  SELF_Demux/11(heading [deg]) -> Terminator_11/1
  SELF_Demux/12(yaw rate [deg/s]) -> Terminator_12/1

== system paper1_cs/Audi_A8_Sedan_3 ==
  SELF_Audi_A8_Sedan_3 : Inport  Tag=inport/SelfPort  OutDataTypeStr=Bus: PRESCAN_SELFSENSORDATA  PortDimensions=1  SampleTime=1/20  BusOutputAsStruct=on
  Dynamics_UserSpecified : Subsystem  Tag=UserSpecified_Subsys  Description=..\..\..\DynamicMode\Extensions\Simulink\CarSim_VehicleDynamics.mdl  mask(User specified subsystem){update=off, sourcefilename=..\..\..\DynamicMode\Extensions\Simulink\CarSim_VehicleDynamics.mdl}
      mask prompts: update "Update (default: not checked)"; sourcefilename "Source file name"
      mask help:
      | A User-specified model may be selected as Controller or Dynamics of the vehicle. PreScan will copy the contents of the User-specified model into the user-specified model block.
      |
      | If update checkbox is checked the current user-specified model block will be deleted and will be REPLACED by (new) user specified model blocks. So, the current user specified model elements will be lost.
      |
      | Warning: If a new user-specified model is selected in the GUI, the user-specified model will be replaced.
      settings: DeleteFcn=PreScanBlockDeleteFcn;
      mask Help: eval('openHelp(227)')
      mask Display: userSpecifiedDynamics_mask_display();
  SELF_Demux : Subsystem  Tag=demux/SelfPort  mask(PreScan Demux Block:){}
      mask help:
      | The SELF port shows (state) information of the actor itself. The outputs are position in the experiment's axis system and the GPS coordinates, and the object's absolute velocity and compass heading.
      |
      | For more information, please click Help.
      settings: DeleteFcn=PreScanBlockDeleteFcn;
      mask Help: eval('openHelp(462)')
      mask Display:
      | port_label('output',1,'x [m]')
      | port_label('output',2,'y [m]')
      | port_label('output',3,'z [m]','texmode','on')
      | port_label('output',4,'Rotx [deg]','texmode','on')
      | port_label('output',5,'Roty [deg]','texmode','on')
      | port_label('output',6,'Rotz [deg]','texmode','on')
      | port_label('output',7,'GPS lat [deg]','texmode','on')
      | port_label('output',8,'GPS long [deg]','texmode','on')
      | port_label('output',9,'GPS alt [m]','texmode','on')
      | port_label('output',10,'Velocity [m/s]')
      | port_label('output',11,'Heading [deg]')
      | port_label('output',12,'Yaw rate [deg/s]')
  STATE_Audi_A8_Sedan_3 : Subsystem  Tag=mux/StatePort  Priority=0  LoadFcn=load PrescanStateActuatorData  mask(PreScan Sink Block: State){x0=80, y0=85, z0=0.55, Roll0=0, Pitch0=0, Yaw0=0, TimeStep=1/20}
      mask prompts: x0 "Ini x-position VEHICLE wrt GLOBAL axis system [m]"; y0 "Ini y-position VEHICLE wrt GLOBAL axis system [m]"; z0 "Ini z-position VEHICLE wrt GLOBAL axis system [m]"; Roll0 "Ini roll-angle BODY wrt VEHICLE axis system [deg]"; Pitch0 "Ini pitch-angle BODY wrt VEHICLE axis system [deg]"; Yaw0 "Ini yaw-angle VEHICLE wrt GLOBAL axis system [deg]"; TimeStep "Auto-Assigned: Upload Period [s]"
      mask help:
      | The Actor State contains a vector signal of size (9x1), containing the following signals:
      |
      | -  Position                  (x,y,z)                                     [m]
      | -  Velocity                  (vx,vy,vz)                               [m/s]
      | -  Angles                    (Roll, Pitch, Yaw)                   [rad]
      |
      | The Actor state is defined in the global axis system.
      | The state is superponed on the Initial position defined in the GUI.
      |
      | For more information, please click Help.
      settings: DeleteFcn=PreScanBlockDeleteFcn;
      mask Help: eval('openHelp(222)')
      mask Display: image(imread('State.png'))
  STATE_Audi_A8_Sedan_3_rc : RateTransition  Tag=mux_rc/StatePort  OutPortSampleTimeOpt=Inherit
  Terminator_{1..12} (12 alike) : Terminator
  STATE_Audi_A8_Sedan_3_bus : Outport  Tag=outport/StatePort  OutDataTypeStr=Bus: PRESCAN_STATEACTUATORDATA  PortDimensions=1  SampleTime=1/20
  wires:
  STATE_Audi_A8_Sedan_3_rc/1 -> STATE_Audi_A8_Sedan_3_bus/1
  STATE_Audi_A8_Sedan_3/1(StateBus) -> STATE_Audi_A8_Sedan_3_rc/1
  SELF_Audi_A8_Sedan_3/1 -> SELF_Demux/1(SELF)
  Dynamics_UserSpecified/1(State) -> STATE_Audi_A8_Sedan_3/1(State)
  SELF_Demux/1(x [m]) -> Terminator_1/1
  SELF_Demux/2(y [m]) -> Terminator_2/1
  SELF_Demux/3(z [m]) -> Terminator_3/1
  SELF_Demux/4(rotx [deg]) -> Terminator_4/1
  SELF_Demux/5(roty [deg]) -> Terminator_5/1
  SELF_Demux/6(rotz [deg]) -> Terminator_6/1
  SELF_Demux/7(GPS lat [deg]) -> Terminator_7/1
  SELF_Demux/8(GPS long [deg]) -> Terminator_8/1
  SELF_Demux/9(GPS alt [m]) -> Terminator_9/1
  SELF_Demux/10(velocity [m/s]) -> Terminator_10/1
  SELF_Demux/11(heading [deg]) -> Terminator_11/1
  SELF_Demux/12(yaw rate [deg/s]) -> Terminator_12/1

== system paper1_cs/Audi_A8_Sedan_4 ==
  SELF_Audi_A8_Sedan_4 : Inport  Tag=inport/SelfPort  OutDataTypeStr=Bus: PRESCAN_SELFSENSORDATA  PortDimensions=1  SampleTime=1/20  BusOutputAsStruct=on
  Dynamics_UserSpecified : Subsystem  Tag=UserSpecified_Subsys  Description=..\..\..\DynamicMode\Extensions\Simulink\CarSim_VehicleDynamics.mdl  mask(User specified subsystem){update=off, sourcefilename=..\..\..\DynamicMode\Extensions\Simulink\CarSim_VehicleDynamics.mdl}
      mask prompts: update "Update (default: not checked)"; sourcefilename "Source file name"
      mask help:
      | A User-specified model may be selected as Controller or Dynamics of the vehicle. PreScan will copy the contents of the User-specified model into the user-specified model block.
      |
      | If update checkbox is checked the current user-specified model block will be deleted and will be REPLACED by (new) user specified model blocks. So, the current user specified model elements will be lost.
      |
      | Warning: If a new user-specified model is selected in the GUI, the user-specified model will be replaced.
      settings: DeleteFcn=PreScanBlockDeleteFcn;
      mask Help: eval('openHelp(227)')
      mask Display: userSpecifiedDynamics_mask_display();
  SELF_Demux : Subsystem  Tag=demux/SelfPort  mask(PreScan Demux Block:){}
      mask help:
      | The SELF port shows (state) information of the actor itself. The outputs are position in the experiment's axis system and the GPS coordinates, and the object's absolute velocity and compass heading.
      |
      | For more information, please click Help.
      settings: DeleteFcn=PreScanBlockDeleteFcn;
      mask Help: eval('openHelp(462)')
      mask Display:
      | port_label('output',1,'x [m]')
      | port_label('output',2,'y [m]')
      | port_label('output',3,'z [m]','texmode','on')
      | port_label('output',4,'Rotx [deg]','texmode','on')
      | port_label('output',5,'Roty [deg]','texmode','on')
      | port_label('output',6,'Rotz [deg]','texmode','on')
      | port_label('output',7,'GPS lat [deg]','texmode','on')
      | port_label('output',8,'GPS long [deg]','texmode','on')
      | port_label('output',9,'GPS alt [m]','texmode','on')
      | port_label('output',10,'Velocity [m/s]')
      | port_label('output',11,'Heading [deg]')
      | port_label('output',12,'Yaw rate [deg/s]')
  STATE_Audi_A8_Sedan_4 : Subsystem  Tag=mux/StatePort  Priority=0  LoadFcn=load PrescanStateActuatorData  mask(PreScan Sink Block: State){x0=60, y0=85, z0=0.55, Roll0=0, Pitch0=0, Yaw0=0, TimeStep=1/20}
      mask prompts: x0 "Ini x-position VEHICLE wrt GLOBAL axis system [m]"; y0 "Ini y-position VEHICLE wrt GLOBAL axis system [m]"; z0 "Ini z-position VEHICLE wrt GLOBAL axis system [m]"; Roll0 "Ini roll-angle BODY wrt VEHICLE axis system [deg]"; Pitch0 "Ini pitch-angle BODY wrt VEHICLE axis system [deg]"; Yaw0 "Ini yaw-angle VEHICLE wrt GLOBAL axis system [deg]"; TimeStep "Auto-Assigned: Upload Period [s]"
      mask help:
      | The Actor State contains a vector signal of size (9x1), containing the following signals:
      |
      | -  Position                  (x,y,z)                                     [m]
      | -  Velocity                  (vx,vy,vz)                               [m/s]
      | -  Angles                    (Roll, Pitch, Yaw)                   [rad]
      |
      | The Actor state is defined in the global axis system.
      | The state is superponed on the Initial position defined in the GUI.
      |
      | For more information, please click Help.
      settings: DeleteFcn=PreScanBlockDeleteFcn;
      mask Help: eval('openHelp(222)')
      mask Display: image(imread('State.png'))
  STATE_Audi_A8_Sedan_4_rc : RateTransition  Tag=mux_rc/StatePort  OutPortSampleTimeOpt=Inherit
  Terminator_{1..12} (12 alike) : Terminator
  STATE_Audi_A8_Sedan_4_bus : Outport  Tag=outport/StatePort  OutDataTypeStr=Bus: PRESCAN_STATEACTUATORDATA  PortDimensions=1  SampleTime=1/20
  wires:
  STATE_Audi_A8_Sedan_4_rc/1 -> STATE_Audi_A8_Sedan_4_bus/1
  STATE_Audi_A8_Sedan_4/1(StateBus) -> STATE_Audi_A8_Sedan_4_rc/1
  SELF_Audi_A8_Sedan_4/1 -> SELF_Demux/1(SELF)
  Dynamics_UserSpecified/1(State) -> STATE_Audi_A8_Sedan_4/1(State)
  SELF_Demux/1(x [m]) -> Terminator_1/1
  SELF_Demux/2(y [m]) -> Terminator_2/1
  SELF_Demux/3(z [m]) -> Terminator_3/1
  SELF_Demux/4(rotx [deg]) -> Terminator_4/1
  SELF_Demux/5(roty [deg]) -> Terminator_5/1
  SELF_Demux/6(rotz [deg]) -> Terminator_6/1
  SELF_Demux/7(GPS lat [deg]) -> Terminator_7/1
  SELF_Demux/8(GPS long [deg]) -> Terminator_8/1
  SELF_Demux/9(GPS alt [m]) -> Terminator_9/1
  SELF_Demux/10(velocity [m/s]) -> Terminator_10/1
  SELF_Demux/11(heading [deg]) -> Terminator_11/1
  SELF_Demux/12(yaw rate [deg/s]) -> Terminator_12/1
